simulink library "commblkcod2"  (Simulink 6.0)
settings: Solver=ode45  SolverMode=SingleTasking  StartTime=0.0  StopTime=10.0  RelTol=1e-3
undefined symbols (not defined in the file or in its folder): a, b, G, gfprimfd, k, n, rsgenpoly
libraries: simulink x17, dspsigattribs x17, commblksprivate x6, commutil2 x4, dspmtrx3 x2, commblkcod2 x2
settings Model: RequirementInfo=9  CovMetricSettings=d  Creator=mikem  LastModifiedBy=cvora  ExtModeAutoUpdateStatusClock=off  ProdHWDeviceType=Specified
settings DataIOCC: SignalLoggingName=logsOut
settings OptimizationCC: BooleanDataType=off
settings DebuggingCC: CheckExecutionContextPreStartOutputMsg=on  CheckExecutionContextRuntimeOutputMsg=on  SolverPrmCheckMsg=none
settings HardwareCC: ProdBitPerShort=32  ProdBitPerInt=16  ProdHWDeviceType=Specified  TargetUnknown=on
settings SFSimCC: SFSimApplyToAllLibs=on  SFSimBuildMode=Incremental

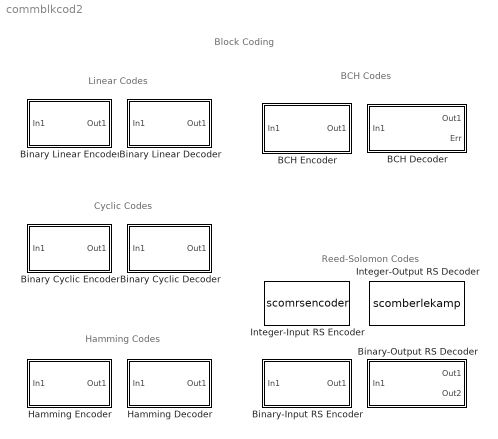
== system commblkcod2 ==
  note: Cyclic Codes
  note: Hamming Codes
  note: BCH Codes
  note: Reed-Solomon Codes
  note: Linear Codes
  note: Block Coding
  BCH Decoder : Subsystem  PropExecContextAcrossSSBoundary=on  mask(BCH Decoder){n=15, k=5, showNumErr=on}
      mask prompts: showNumErr "Output number of corrected errors"
      mask help:
      | Decode a BCH codeword with message length K and codeword length N. N must have the form 2^M-1, where 3 <= M <= 9 .  The values of N and K must produce a valid narrow-sense BCH codeword.
      |
      | The input must contain exactly N elements. The input must be a frame-based column vector.
      mask init:
      | params = commblksbchdec(n,k, showNumErr);
      mask Help: helpview(commbhelp)
      mask Display:
      | plot(0,0,100,100,[5 15 15 5 15 15 5 5 15 15 20 15 75 75 85 75 75 15 75 75 85 85 95 95 85 85 95],[75 75 85 85 85 65 65 95 95 83 80 77 77 73 80 87 83 83 83 87 80 90 90 70 70 80 80]);disp('BCH de');
      | port_label('output',params.portnum, params.portlabel);
  BCH Encoder : Subsystem  PropExecContextAcrossSSBoundary=on  mask(BCH Encoder){n=15, k=5}
      mask help:
      | Create a BCH code with message length K and codeword length N. N must have the form 2^M-1, where 3 <= M <= 9.  The values of N and K must produce a valid narrow-sense BCH codeword.
      |
      | The input must contain exactly K elements. The input must be a frame-based column vector.
      mask init:
      | genpoly = bchgenpoly(n,k);
      | [h, gen] = cyclgen(n,double(genpoly.x));
      | gen1 =[ gen(:,n-k+1:end) gen(:,1:n-k) ];
      mask Help: helpview(commbhelp)
      mask Display: plot(0,0,100,100,[05 15 15 05 05 15 15 15  15 20 15 75 75 85 75 75 15 75 75  85 85 95 95 85 85 95 85 85 95],[80 80 90 90 70 70 90 80  83 80 77 77 73 80 87 83 83 83 87  80 95 95 65 65 85 85 85 75 75]);disp('BCH en')
  Binary Cyclic Decoder : Subsystem  PropExecContextAcrossSSBoundary=on  mask(Binary Cyclic Decoder){n=7, p=4}
      mask prompts: n "Codeword length N:"; p "Message length K, or generator polynomial:"
      mask help:
      | Recover a message vector from a codeword vector of a binary systematic cyclic code.  The message is of length K and the codeword is of length N, where N has the form 2^M-1, for some integer M greater than or equal to 3.
      |
      | The input must contain exactly N elements.  If it is frame-based, then it must be a column vector.
      mask init:
      | m=log2(n+1); if ~isequal(floor(m),m) | n<3,error('N must have the form 2^M-1 for some integer M greater than 2.');end;
      | evalc('if isequal(length(p),1),p=cyclpoly(n,p,''min'');if isempty(p), error(''No cyclic code exists for specified values of N and K.''); end; end;[H,G]=cyclgen(n,p);trt=syndtable(H);');[k,n]=size(G);
      mask Help: helpview(commbhelp)
      mask Display:
      | plot(0,0,100,100,[5 15 15 5 15 15 5 5 15 15 20 15 75 75 85 75 75 15 75 75 85 85 95 95 85 85 95],[75 75 85 85 85 65 65 95 95 83 80 77 77 73 80 87 83 83 83 87 80 90 90 70 70 80 80]);
      | disp('Cyclic de')
  Binary Cyclic Encoder : Subsystem  PropExecContextAcrossSSBoundary=on  mask(Binary Cyclic Encoder){n=7, p=4}
      mask prompts: n "Codeword length N:"; p "Message length K, or generator polynomial:"
      mask help:
      | Create a systematic cyclic code with message length K and codeword length N.  The number N must have the form 2^M-1, where M is an integer greater than or equal to 3.
      |
      | The input must contain exactly K elements.  If it is frame-based, then it must be a column vector.
      mask init:
      | m=log2(n+1); if ~isequal(floor(m),m) | n<3,error('N must have the form 2^M-1 for some integer M >= 3.');end;evalc('if length(p)==1,p=cyclpoly(n,p,''min''); if isempty(p),error(''No cyclic code exists for specified values of N and K.'');end;end;  k=n-length(p)+1; [h,G]=cyclgen(n, p);');
      mask Help: helpview(commbhelp)
      mask Display:
      | plot(0,0,100,100,[05 15 15 05 05 15 15 15  15 20 15 75 75 85 75 75 15 75 75  85 85 95 95 85 85 95 85 85 95],[80 80 90 90 70 70 90 80  83 80 77 77 73 80 87 83 83 83 87  80 95 95 65 65 85 85 85 75 75]);
      | disp('Cyclic en')
  Binary Linear Decoder : Subsystem  PropExecContextAcrossSSBoundary=on  mask(Binary Linear Decoder){G=[[1 1 0; 0 1 1; 1 1 1;1 0 1] eye(4)], trt=0}
      mask prompts: G "Generator matrix (binary K-by-N matrix):"; trt "Decoding table (0 for table corresponding to Generator matrix):"
      mask help:
      | Recover a binary message vector from a binary codeword vector of a linear block code.  The message is of length K and the codeword is of length N, where K and N are the number of rows and columns of the generator matrix respectively.  The number N must have the form 2^M-1, for some integer M greater than or equal to 3.
      |
      | The decoder assumes that the encoder's generator matrix has the standard systematic form [P I].  In other words, the input codewords must contain parity-check bits followed by message bits.
      |
      | The input must contain exactly N elements.  If it is frame-based, then it must be a column vector.
      mask init:
      | [k,n]=size(G);  if k>=n | ~isequal(G(:,n-k+1:n),eye(k)), error('The generator matrix must have the standard systematic form [P I].'); end;
      | H=gen2par(G);if trt==0,evalc('trt=syndtable(H);');end;
      mask Help: helpview(commbhelp)
      mask Display:
      | plot(0,0,100,100,[5 15 15 5 15 15 5 5 15 15 20 15 75 75 85 75 75 15 75 75 85 85 95 95 85 85 95],[75 75 85 85 85 65 65 95 95 83 80 77 77 73 80 87 83 83 83 87 80 90 90 70 70 80 80]);
      | disp('Linear de')
  Binary Linear Encoder : Subsystem  PropExecContextAcrossSSBoundary=on  mask(Binary Linear Encoder){G=[[1 1 0; 0 1 1; 1 1 1; 1 0 1] eye(4)]}
      mask prompts: G "Generator matrix (binary K-by-N matrix):"
      mask help:
      | Create a binary linear block code with message length K and codeword length N, where K and N are the number of rows and columns of the generator matrix respectively.
      |
      | To use the Binary Linear Decoder block at the decoder side, provide a generator matrix in the standard systematic form [P I].
      |
      | The input must contain exactly K elements.  If it is frame-based, then it must be a column vector.
      mask init:
      | [k n]=size(G);
      mask Help: helpview(commbhelp)
      mask Display:
      | plot(0,0,100,100,[05 15 15 05 05 15 15 15  15 20 15 75 75 85 75 75 15 75 75  85 85 95 95 85 85 95 85 85 95],[80 80 90 90 70 70 90 80  83 80 77 77 73 80 87 83 83 83 87  80 95 95 65 65 85 85 85 75 75]);
      | disp('Linear en')
  Binary-Input RS Encoder : Subsystem  PropExecContextAcrossSSBoundary=on  mask(Binary-Input RS Encoder){n=7, k=3, specPrimPoly=off, primPoly=[1 0 1 1], specGenPoly=off, genPoly=rsgenpoly(7,3)}
      mask prompts: n "Codeword length N:"; k "Message length K:"; specPrimPoly "Specify primitive polynomial"; primPoly "Primitive polynomial:"; specGenPoly "Specify generator polynomial"; genPoly "Generator polynomial:"
      mask help:
      | Encode the message in the input vector using an (N,K) Reed-Solomon encoder with the narrow-sense generator polynomial.  The input must be a frame-based column vector with an integer multiple of K*ceil(log2(N+1)) bits.  Each group of K*ceil(log2(N+1)) input bits represents one message word to be encoded.
      |
      | The optional 'Primitive polynomial' parameter is a row vector that represents the binary coefficients of the primitive polynomial in order of descending powers.  When such a user-defined Primitive polynomial is provided, the number of input bits must be an integer multiple of K times the order of the Primitive polynomial instead.
      |
      | The optional 'Generator polynomial' parameter is a row vector that represents the coefficients of the generator polynomial in order of descending powers.  Each coefficient is an element of the Galois field defined by the primitive polynomial.
      mask init:
      | [eStr,params]=commblkrsencbin(gcb, 'init');
      | if(eStr.ecode==1)
      |     error(eStr.emsg);
      | elseif(eStr.ecode==2)
      |     warning(eStr.emsg);
      | end;
      mask Help: helpview(commbhelp)
      mask CallbackString: ||commblkrsencbin(gcb,'cbSpecPrimPoly');||commblkrsencbin(gcb,'cbSpecGenPoly');|
      mask Display:
      | plot(0,0,100,100,[05 15 15 05 05 15 15 15  15 20 15 75 75 85 75 75 15 75 75  85 85 95 95 85 85 95 85 85 95],[80 80 90 90 70 70 90 80  83 80 77 77 73 80 87 83 83 83 87  80 95 95 65 65 85 85 85 75 75]);
      | disp('\nBinary Input\nRS Encoder')
  Binary-Output RS Decoder : Subsystem  PropExecContextAcrossSSBoundary=on  mask(Binary-Output RS Decoder){n=7, k=3, specPrimPoly=off, primPoly=[1 0 1 1], specGenPoly=off, genPoly=rsgenpoly(7,3), showNumErr=on}
      mask prompts: n "Codeword length N:"; k "Message length K:"; specPrimPoly "Specify primitive polynomial"; primPoly "Primitive polynomial:"; specGenPoly "Specify generator polynomial"; genPoly "Generator polynomial:"; showNumErr "Output number of corrected errors"
      mask help:
      | Attempt to decode the input received signal using an (N,K) Reed-Solomon decoder with the narrow-sense generator polynomial.  The input must be a frame-based column vector with an integer multiple of N*ceil(log2(N+1)) bits.  Each group of N*ceil(log2(N+1)) input bits represents one received word to be decoded.
      |
      | The optional 'Primitive polynomial' parameter is a row vector that represents the binary coefficients of the primitive polynomial in order of descending powers.  When such a user-defined Primitive polynomial is provided, the number of input bits must be an integer multiple of N times the order of the Primitive polynomial instead.
      |
      | The optional 'Generator polynomial' parameter is a row vector that represents the coefficients of the generator polynomial in order of descending powers.  Each coefficient is an element of the Galois field defined by the primitive polynomial.
      |
      | The number of corrected errors can be sent to a second output port by checking the 'Output number of corrected errors' check box.  A decoding failure occurs when a certain received word in the input contains more than (N-K)/2 symbol errors.  This is indicated by a value of -1 in the corresponding position in the second output vector.
      mask init:
      | [eStr,params]=commblkrsdecbin(gcb, 'init');
      | if(eStr.ecode==1)
      |     error(eStr.emsg);
      | elseif(eStr.ecode==2)
      |     warning(eStr.emsg);
      | end;
      mask Help: helpview(commbhelp)
      mask CallbackString: ||commblkrsdecbin(gcb,'cbSpecPrimPoly');||commblkrsdecbin(gcb,'cbSpecGenPoly');||commblkrsdecbin(gcb,'cbShowNumErr');
      mask Display:
      | plot(0,0,100,100,[5 15 15 5 15 15 5 5 15 15 20 15 75 75 85 75 75 15 75 75 85 85 95 95 85 85 95],[75 75 85 85 85 65 65 95 95 83 80 77 77 73 80 87 83 83 83 87 80 90 90 70 70 80 80]);
      | disp('\nBinary Output\nRS Decoder')
      | text(params.x,params.y,params.portlabel)
  Hamming Decoder : Subsystem  PropExecContextAcrossSSBoundary=on  mask(Hamming Decoder){n=7, k=gfprimfd(3,'min')}
      mask prompts: n "Codeword length N:"; k "Message length K, or M-degree primitive polynomial:"
      mask help:
      | Recover a binary message vector from a binary Hamming codeword vector.  The message is of length K and the codeword is of length N, where N has the form 2^M-1, for some integer M greater than or equal to 3.  K must equal N-M.
      |
      | The input must contain exactly N elements.  If it is frame-based, then it must be a column vector.
      mask init:
      | if length(k)>1,p=k;k=n-length(p)+1;
      | else,evalc('p=gfprimdf(n-k);');end;
      | m=log2(n+1);if ~isequal(floor(m),m) | ~isequal(n-k,m), error('N must have the form 2^M-1 where M is an integer >=3.  K must equal N-M.');end;
      | evalc('[H,G]=hammgen(n-k,p);trt=syndtable(H);');[a,b]=size(G);
      mask Help: helpview(commbhelp)
      mask Display: plot(0,0,100,100,[1 3 3 1 3 3 1 1 3 3 4 3 15 15 17 15 15 3 15 15 17 17 19 19 17 17 19]*5,[-5 -5 5 5 5 -15 -15 15 15 3 0 -3 -3 -7 0 7 3 3 3 7 0 10 10 -10 -10 0 0]+80);disp('Hamming de')
  Hamming Encoder : Subsystem  PropExecContextAcrossSSBoundary=on  mask(Hamming Encoder){n=7, k=gfprimfd(3,'min')}
      mask prompts: n "Codeword length N:"; k "Message length K, or M-degree primitive polynomial:"
      mask help:
      | Create a Hamming code with message length K and codeword length N.  The number N must have the form 2^M-1, where M is an integer greater than or equal to 3.  K must equal N-M.
      |
      | The input must contain exactly K elements.  If it is frame-based, then it must be a column vector.
      mask init:
      | if length(k)>1, p=k; k=n-length(k)+1;
      | else, evalc('p=gfprimdf(n-k);'); end;
      | m=log2(n+1);if ~isequal(floor(m),m) | ~isequal(n-k,m), error('N must have the form 2^M-1 where M is an integer >=3.  K must equal N-M.');end;
      | evalc('[h,G]=hammgen(n-k,p);');
      mask Help: helpview(commbhelp)
      mask Display: plot(0,0,100,100,[1 3 3 1 1 3 3 3 3 4 3 15 15 17 15 15 3 15 15 17 17 19 19 17 17 19 17 17 19]*5,[0 0 10 10 -10 -10 10 0 3 0 -3 -3 -7 0 7 3 3 3 7 0 15 15 -15 -15 5 5 5 -5 -5]+80);disp('Hamming en')
  Integer-Input RS Encoder : S-Function  FunctionName=scomrsencoder  Parameters=n, k, params.m, params.primPoly, params.genPoly, params.shortened  mask(Integer-Input RS Encoder){n=7, k=3, specPrimPoly=off, primPoly=[1 0 1 1], specGenPoly=off, genPoly=rsgenpoly(7,3)}
      mask prompts: n "Codeword length N:"; k "Message length K:"; specPrimPoly "Specify primitive polynomial"; primPoly "Primitive polynomial:"; specGenPoly "Specify generator polynomial"; genPoly "Generator polynomial:"
      mask help:
      | Encode the message in the input vector using an (N,K) Reed-Solomon encoder with the narrow-sense generator polynomial.  The input must be a frame-based column vector with an integer multiple of K elements.  Each group of K input elements represents one message word to be encoded.  Each symbol must have ceil(log2(N+1)) bits.
      |
      | The optional 'Primitive polynomial' parameter is a row vector that represents the binary coefficients of the primitive polynomial in order of descending powers.  When such a user-defined Primitive polynomial is provided, the number of bits in each input symbol must equal the order of the Primitive polynomial instead.
      |
      | The optional 'Generator polynomial' parameter is a row vector that represents the coefficients of the generator polynomial in order of descending powers.  Each coefficient is an element of the Galois field defined by the primtive polynomial.
      mask init:
      | [eStr,params]=commblkrsencoder(gcb, 'init');
      | if(eStr.ecode==1)
      |     error(eStr.emsg);
      | elseif(eStr.ecode==2)
      |     warning(eStr.emsg);
      | end;
      mask Help: helpview(commbhelp)
      mask CallbackString: ||commblkrsencoder(gcb,'cbSpecPrimPoly');||commblkrsencoder(gcb,'cbSpecGenPoly');|
      mask Display:
      | plot(0,0,100,100,[05 15 15 05 05 15 15 15  15 20 15 75 75 85 75 75 15 75 75  85 85 95 95 85 85 95 85 85 95],[80 80 90 90 70 70 90 80  83 80 77 77 73 80 87 83 83 83 87  80 95 95 65 65 85 85 85 75 75]);
      | disp('\nRS Encoder')
  Integer-Output RS Decoder : S-Function  FunctionName=scomberlekamp  Parameters=n, k, params.m, params.t, params.primPoly, params.b, params.shortened, showNumErr  mask(Integer-Output RS Decoder){n=7, k=3, specPrimPoly=off, primPoly=[1 0 1 1], specGenPoly=off, genPoly=rsgenpoly(7,3), showNumErr=on}
      mask prompts: n "Codeword length N:"; k "Message length K:"; specPrimPoly "Specify primitive polynomial"; primPoly "Primitive polynomial:"; specGenPoly "Specify generator polynomial"; genPoly "Generator polynomial:"; showNumErr "Output number of corrected errors"
      mask help:
      | Attempt to decode the input received signal using an (N,K) Reed-Solomon decoder with the narrow-sense generator polynomial.  The input must be a frame-based column vector with an integer multiple of N elements.  Each group of N input elements represents one received word to be decoded.  Each symbol must have ceil(log2(N+1)) bits.
      |
      | The optional 'Primitive polynomial' parameter is a row vector that represents the binary coefficients of the primitive polynomial in order of descending powers.  When such a user-defined Primitive polynomial is provided, the number of bits in each input symbol must equal the order of the Primitive polynomial instead.
      |
      | The optional 'Generator polynomial' parameter is a row vector that represents the coefficients of the generator polynomial in order of descending powers.  Each coefficient is an element of the Galois field defined by the primitive polynomial.
      |
      | The number of corrected errors can be sent to a second output port by checking the 'Output number of corrected errors' check box.  A decoding failure occurs when a certain word in the input contains more than (N-K)/2 errors.  This is indicated by a value of -1 in the corresponding position in the second output vector.
      mask init:
      | [eStr,params]=commblkrsdecoder(gcb, 'init');
      | if(eStr.ecode==1)
      |     error(eStr.emsg);
      | elseif(eStr.ecode==2)
      |     warning(eStr.emsg);
      | end;
      mask Help: helpview(commbhelp)
      mask CallbackString: ||commblkrsdecoder(gcb,'cbSpecPrimPoly');||commblkrsdecoder(gcb,'cbSpecGenPoly');||
      mask Display:
      | plot(0,0,100,100,[5 15 15 5 15 15 5 5 15 15 20 15 75 75 85 75 75 15 75 75 85 85 95 95 85 85 95],[75 75 85 85 85 65 65 95 95 83 80 77 77 73 80 87 83 83 83 87 80 90 90 70 70 80 80]);
      | disp('\nRS Decoder')
      | port_label('output',params.portnum,params.portlabel);

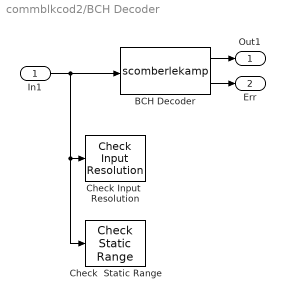
== system commblkcod2/BCH Decoder ==
  In1 : Inport  LatchInput=off
  BCH Decoder : S-Function  FunctionName=scomberlekamp  Parameters=n,k,params.m, params.t,params.poly,1,0,1
  Check  Static Range : simulink/Model Verification/Check  Static Range  Description=0 <= u <= 1  max=1  max_included=on  min=0  min_included=on  enabled=on  callback=error('Input must be 0 or 1')  stopWhenAssertionFail=on  export=off  icon=graphic
  Check Input  Resolution : simulink/Model Verification/Check Input  Resolution  Description=-Inf < u < +Inf  resolution=1  enabled=on  callback=error('Input must be 0 or 1')  stopWhenAssertionFail=on  export=off
  Out1 : Outport
  Err : Outport  Port=2
  wires:
  BCH Decoder/2 -> Err/1
  BCH Decoder/1 -> Out1/1
  In1/1 -> BCH Decoder/1, Check Input  Resolution/1, Check  Static Range/1

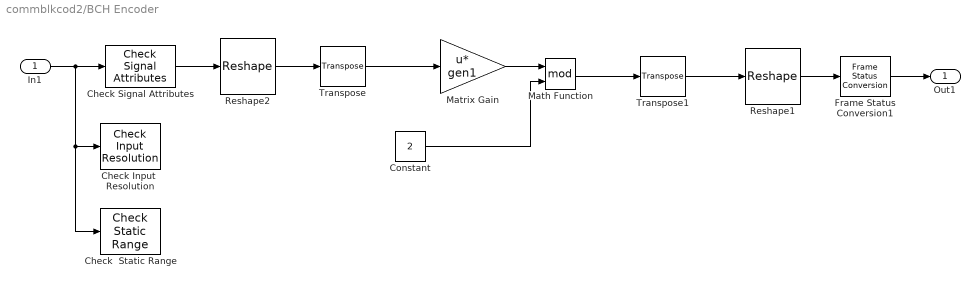
== system commblkcod2/BCH Encoder ==
  In1 : Inport  LatchInput=off
  Check  Static Range : simulink/Model Verification/Check  Static Range  Description=0 <= u <= 1  max=1  max_included=on  min=0  min_included=on  enabled=on  callback=error('Input must be 0 or 1')  stopWhenAssertionFail=on  export=off  icon=graphic
  Check Input  Resolution : simulink/Model Verification/Check Input  Resolution  Description=-Inf < u < +Inf  resolution=1  enabled=on  callback=error('Input must be 0 or 1')  stopWhenAssertionFail=on  export=off
  Check Signal Attributes : dspsigattribs/Check Signal Attributes  SigAttribCheckMethod=Does not match attributes exactly  Complexity=Real  Frame=Frame-based  DimsCheckMethod=Is...  Dimensions=Column vector (2-D)  DatatypeCheckMethod=Ignore  DatatypeGeneral=Boolean  DtypeFloatSpecific=Any floating-point  DtypeFixedSpecific=Any fixed-point  DtypeIntSpecific=Any integer  SampleMode=Ignore
      settings: AttributesFormatString=\n
  Constant : Constant  Value=2
  Frame Status Conversion1 : dspsigattribs/Frame Status Conversion  growRefPort=off  outframe=Frame-based
      settings: AttributesFormatString=\n
  Math Function : Math  Operator=mod  SaturateOnIntegerOverflow=on
  Matrix Gain : Gain  Gain=gen1  Multiplication=Matrix(u*K)  SaturateOnIntegerOverflow=on
  Reshape1 : simulink/Math Operations/Reshape  OutputDimensionality=Customize  OutputDimensions=[n,1]
  Reshape2 : simulink/Math Operations/Reshape  OutputDimensionality=Customize  OutputDimensions=[k, 1 ]
  Transpose : dspmtrx3/Transpose  Hermitian=off
      settings: AttributesFormatString=\n
  Transpose1 : dspmtrx3/Transpose  Hermitian=off
      settings: AttributesFormatString=\n
  Out1 : Outport
  wires:
  Check Signal Attributes/1 -> Reshape2/1
  Frame Status Conversion1/1 -> Out1/1
  Reshape1/1 -> Frame Status Conversion1/1
  Transpose1/1 -> Reshape1/1
  Transpose/1 -> Matrix Gain/1
  In1/1 -> Check Signal Attributes/1, Check Input  Resolution/1, Check  Static Range/1
  Math Function/1 -> Transpose1/1
  Reshape2/1 -> Transpose/1
  Constant/1 -> Math Function/2
  Matrix Gain/1 -> Math Function/1

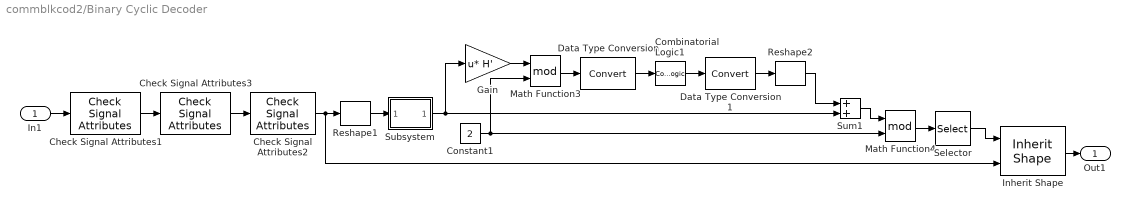
== system commblkcod2/Binary Cyclic Decoder ==
  In1 : Inport  LatchInput=off
  Check Signal Attributes1 : dspsigattribs/Check Signal Attributes  SigAttribCheckMethod=Matches attributes exactly  Complexity=Ignore  Frame=Frame-based  DimsCheckMethod=Is...  Dimensions=Row vector (2-D)  DatatypeCheckMethod=Ignore  DatatypeGeneral=Boolean  DtypeFloatSpecific=Any floating-point  DtypeFixedSpecific=Any fixed-point  DtypeIntSpecific=Any integer  SampleMode=Ignore
  Check Signal Attributes2 : dspsigattribs/Check Signal Attributes  SigAttribCheckMethod=Matches attributes exactly  Complexity=Ignore  Frame=Ignore  DimsCheckMethod=Is...  Dimensions=Full matrix (2-D)  DatatypeCheckMethod=Ignore  DatatypeGeneral=Boolean  DtypeFloatSpecific=Any floating-point  DtypeFixedSpecific=Any fixed-point  DtypeIntSpecific=Any integer  SampleMode=Ignore
  Check Signal Attributes3 : dspsigattribs/Check Signal Attributes  SigAttribCheckMethod=Matches attributes exactly  Complexity=Ignore  Frame=Ignore  DimsCheckMethod=Is...  Dimensions=Scalar (1-D or 2-D)  DatatypeCheckMethod=Ignore  DatatypeGeneral=Boolean  DtypeFloatSpecific=Any floating-point  DtypeFixedSpecific=Any fixed-point  DtypeIntSpecific=Any integer  SampleMode=Ignore
  Combinatorial Logic1 : CombinatorialLogic  TruthTable=trt
  Constant1 : Constant  Value=2
  Data Type Conversion : DataTypeConversion  OutDataTypeMode=boolean  SaturateOnIntegerOverflow=on  RndMeth=Zero
  Data Type Conversion1 : DataTypeConversion  OutDataTypeMode=double  SaturateOnIntegerOverflow=on  RndMeth=Zero
  Gain : Gain  Gain=H'  Multiplication=Matrix(u*K)  SaturateOnIntegerOverflow=on
  Inherit Shape : commblksprivate/Inherit Shape
  Math Function3 : Math  Operator=mod  SaturateOnIntegerOverflow=on
  Math Function4 : Math  Operator=mod  SaturateOnIntegerOverflow=on
  Reshape1 : simulink/Math Operations/Reshape  OutputDimensionality=Row vector  OutputDimensions=[1,1]
  Reshape2 : simulink/Math Operations/Reshape  OutputDimensionality=Row vector  OutputDimensions=[1,1]
  Selector : Selector  Elements=[n-k+1:n]  InputPortWidth=n
  Subsystem : Subsystem  AncestorBlock=commblkcod2/Binary Linear Decoder/Subsystem  PropExecContextAcrossSSBoundary=on
  Sum1 : Sum  SaturateOnIntegerOverflow=on  InputSameDT=on
  Out1 : Outport
  wires:
  Check Signal Attributes1/1 -> Check Signal Attributes3/1
  Check Signal Attributes2/1 -> Reshape1/1, Inherit Shape/2
  Inherit Shape/1 -> Out1/1
  In1/1 -> Check Signal Attributes1/1
  Gain/1 -> Math Function3/1
  Combinatorial Logic1/1 -> Data Type Conversion1/1
  Sum1/1 -> Math Function4/1
  Math Function4/1 -> Selector/1
  Math Function3/1 -> Data Type Conversion/1
  Constant1/1 -> Math Function3/2, Math Function4/2
  Selector/1 -> Inherit Shape/1
  Reshape1/1 -> Subsystem/1(In1)
  Subsystem/1(Out1) -> Gain/1, Sum1/2
  Check Signal Attributes3/1 -> Check Signal Attributes2/1
  Reshape2/1 -> Sum1/1
  Data Type Conversion1/1 -> Reshape2/1
  Data Type Conversion/1 -> Combinatorial Logic1/1

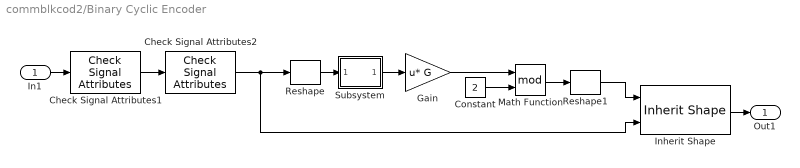
== system commblkcod2/Binary Cyclic Encoder ==
  In1 : Inport  LatchInput=off
  Check Signal Attributes1 : dspsigattribs/Check Signal Attributes  SigAttribCheckMethod=Matches attributes exactly  Complexity=Ignore  Frame=Frame-based  DimsCheckMethod=Is...  Dimensions=Row vector (2-D)  DatatypeCheckMethod=Ignore  DatatypeGeneral=Boolean  DtypeFloatSpecific=Any floating-point  DtypeFixedSpecific=Any fixed-point  DtypeIntSpecific=Any integer  SampleMode=Ignore
  Check Signal Attributes2 : dspsigattribs/Check Signal Attributes  SigAttribCheckMethod=Matches attributes exactly  Complexity=Ignore  Frame=Ignore  DimsCheckMethod=Is...  Dimensions=Full matrix (2-D)  DatatypeCheckMethod=Ignore  DatatypeGeneral=Boolean  DtypeFloatSpecific=Any floating-point  DtypeFixedSpecific=Any fixed-point  DtypeIntSpecific=Any integer  SampleMode=Ignore
  Constant : Constant  Value=2
  Gain : Gain  Gain=G  Multiplication=Matrix(u*K)  SaturateOnIntegerOverflow=on
  Inherit Shape : commblksprivate/Inherit Shape
  Math Function : Math  Operator=mod  SaturateOnIntegerOverflow=on
  Reshape : simulink/Math Operations/Reshape  OutputDimensionality=Row vector  OutputDimensions=[1,1]
  Reshape1 : simulink/Math Operations/Reshape  OutputDimensionality=Column vector  OutputDimensions=[1,1]
  Subsystem : Subsystem  AncestorBlock=commblkcod2/Binary Linear Decoder/Subsystem  PropExecContextAcrossSSBoundary=on
  Out1 : Outport
  wires:
  Constant/1 -> Math Function/2
  Gain/1 -> Math Function/1
  Check Signal Attributes1/1 -> Check Signal Attributes2/1
  Check Signal Attributes2/1 -> Reshape/1, Inherit Shape/2
  Math Function/1 -> Reshape1/1
  Reshape/1 -> Subsystem/1(In1)
  In1/1 -> Check Signal Attributes1/1
  Inherit Shape/1 -> Out1/1
  Subsystem/1(Out1) -> Gain/1
  Reshape1/1 -> Inherit Shape/1

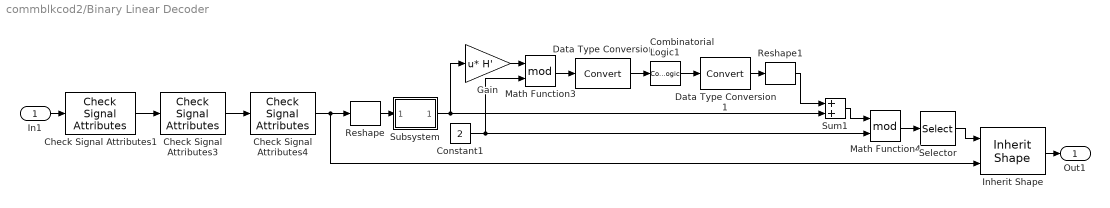
== system commblkcod2/Binary Linear Decoder ==
  In1 : Inport  LatchInput=off
  Check Signal Attributes1 : dspsigattribs/Check Signal Attributes  SigAttribCheckMethod=Matches attributes exactly  Complexity=Ignore  Frame=Frame-based  DimsCheckMethod=Is...  Dimensions=Row vector (2-D)  DatatypeCheckMethod=Ignore  DatatypeGeneral=Boolean  DtypeFloatSpecific=Any floating-point  DtypeFixedSpecific=Any fixed-point  DtypeIntSpecific=Any integer  SampleMode=Ignore
  Check Signal Attributes3 : dspsigattribs/Check Signal Attributes  SigAttribCheckMethod=Matches attributes exactly  Complexity=Ignore  Frame=Ignore  DimsCheckMethod=Is...  Dimensions=Scalar (1-D or 2-D)  DatatypeCheckMethod=Ignore  DatatypeGeneral=Boolean  DtypeFloatSpecific=Any floating-point  DtypeFixedSpecific=Any fixed-point  DtypeIntSpecific=Any integer  SampleMode=Ignore
  Check Signal Attributes4 : dspsigattribs/Check Signal Attributes  SigAttribCheckMethod=Matches attributes exactly  Complexity=Ignore  Frame=Ignore  DimsCheckMethod=Is...  Dimensions=Full matrix (2-D)  DatatypeCheckMethod=Ignore  DatatypeGeneral=Boolean  DtypeFloatSpecific=Any floating-point  DtypeFixedSpecific=Any fixed-point  DtypeIntSpecific=Any integer  SampleMode=Ignore
  Combinatorial Logic1 : CombinatorialLogic  TruthTable=trt
  Constant1 : Constant  Value=2
  Data Type Conversion : DataTypeConversion  OutDataTypeMode=boolean  SaturateOnIntegerOverflow=on  RndMeth=Zero
  Data Type Conversion1 : DataTypeConversion  OutDataTypeMode=double  SaturateOnIntegerOverflow=on  RndMeth=Zero
  Gain : Gain  Gain=H'  Multiplication=Matrix(u*K)  SaturateOnIntegerOverflow=on
  Inherit Shape : commblksprivate/Inherit Shape
  Math Function3 : Math  Operator=mod  SaturateOnIntegerOverflow=on
  Math Function4 : Math  Operator=mod  SaturateOnIntegerOverflow=on
  Reshape : simulink/Math Operations/Reshape  OutputDimensionality=Row vector  OutputDimensions=[1,1]
  Reshape1 : simulink/Math Operations/Reshape  OutputDimensionality=Row vector  OutputDimensions=[1,1]
  Selector : Selector  Elements=[n-k+1:n]  InputPortWidth=n
  Subsystem : Subsystem  AncestorBlock=commblkcod2/Binary Linear Encoder/Subsystem  PropExecContextAcrossSSBoundary=on
  Sum1 : Sum  SaturateOnIntegerOverflow=on  InputSameDT=on
  Out1 : Outport
  wires:
  Gain/1 -> Math Function3/1
  Combinatorial Logic1/1 -> Data Type Conversion1/1
  Sum1/1 -> Math Function4/1
  Math Function4/1 -> Selector/1
  Math Function3/1 -> Data Type Conversion/1
  Constant1/1 -> Math Function4/2, Math Function3/2
  In1/1 -> Check Signal Attributes1/1
  Check Signal Attributes1/1 -> Check Signal Attributes3/1
  Selector/1 -> Inherit Shape/1
  Reshape/1 -> Subsystem/1(In1)
  Subsystem/1(Out1) -> Sum1/2, Gain/1
  Inherit Shape/1 -> Out1/1
  Check Signal Attributes3/1 -> Check Signal Attributes4/1
  Check Signal Attributes4/1 -> Reshape/1, Inherit Shape/2
  Reshape1/1 -> Sum1/1
  Data Type Conversion/1 -> Combinatorial Logic1/1
  Data Type Conversion1/1 -> Reshape1/1

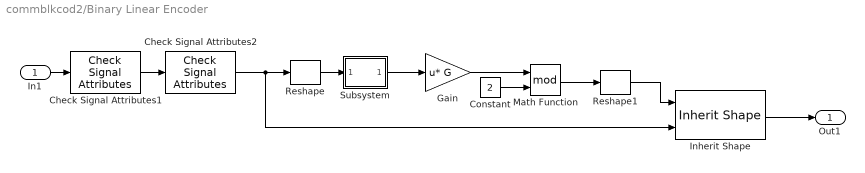
== system commblkcod2/Binary Linear Encoder ==
  In1 : Inport  LatchInput=off
  Check Signal Attributes1 : dspsigattribs/Check Signal Attributes  SigAttribCheckMethod=Matches attributes exactly  Complexity=Ignore  Frame=Frame-based  DimsCheckMethod=Is...  Dimensions=Row vector (2-D)  DatatypeCheckMethod=Ignore  DatatypeGeneral=Boolean  DtypeFloatSpecific=Any floating-point  DtypeFixedSpecific=Any fixed-point  DtypeIntSpecific=Any integer  SampleMode=Ignore
  Check Signal Attributes2 : dspsigattribs/Check Signal Attributes  SigAttribCheckMethod=Matches attributes exactly  Complexity=Ignore  Frame=Ignore  DimsCheckMethod=Is...  Dimensions=Full matrix (2-D)  DatatypeCheckMethod=Ignore  DatatypeGeneral=Boolean  DtypeFloatSpecific=Any floating-point  DtypeFixedSpecific=Any fixed-point  DtypeIntSpecific=Any integer  SampleMode=Ignore
  Constant : Constant  Value=2
  Gain : Gain  Gain=G  Multiplication=Matrix(u*K)  SaturateOnIntegerOverflow=on
  Inherit Shape : commblksprivate/Inherit Shape
  Math Function : Math  Operator=mod  SaturateOnIntegerOverflow=on
  Reshape : simulink/Math Operations/Reshape  OutputDimensionality=Row vector  OutputDimensions=[1,1]
  Reshape1 : simulink/Math Operations/Reshape  OutputDimensionality=Column vector  OutputDimensions=[1,1]
  Subsystem : Subsystem  AncestorBlock=commblkcod2/Binary Linear Decoder/Subsystem  PropExecContextAcrossSSBoundary=on
  Out1 : Outport
  wires:
  Constant/1 -> Math Function/2
  In1/1 -> Check Signal Attributes1/1
  Check Signal Attributes1/1 -> Check Signal Attributes2/1
  Check Signal Attributes2/1 -> Inherit Shape/2, Reshape/1
  Math Function/1 -> Reshape1/1
  Inherit Shape/1 -> Out1/1
  Reshape/1 -> Subsystem/1(In1)
  Gain/1 -> Math Function/1
  Subsystem/1(Out1) -> Gain/1
  Reshape1/1 -> Inherit Shape/1

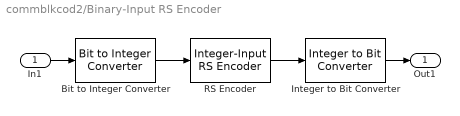
== system commblkcod2/Binary-Input RS Encoder ==
  In1 : Inport  LatchInput=off
  Bit to Integer Converter : commutil2/Bit to Integer Converter  nbits=params.m
  Integer to Bit Converter : commutil2/Integer to Bit Converter  nbits=params.m
  RS Encoder : commblkcod2/Integer-Input RS Encoder  n=n  k=k  specPrimPoly=off  primPoly=primPoly  specGenPoly=off  genPoly=genPoly
  Out1 : Outport
  wires:
  Bit to Integer Converter/1 -> RS Encoder/1
  RS Encoder/1 -> Integer to Bit Converter/1
  Integer to Bit Converter/1 -> Out1/1
  In1/1 -> Bit to Integer Converter/1

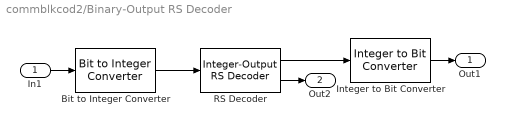
== system commblkcod2/Binary-Output RS Decoder ==
  In1 : Inport  LatchInput=off
  Bit to Integer Converter : commutil2/Bit to Integer Converter  nbits=params.m
  Integer to Bit Converter : commutil2/Integer to Bit Converter  nbits=params.m
  RS Decoder : commblkcod2/Integer-Output RS Decoder  n=n  k=k  specPrimPoly=off  primPoly=primPoly  specGenPoly=off  genPoly=genPoly  showNumErr=on
  Out1 : Outport
  Out2 : Outport  Port=2
  wires:
  In1/1 -> Bit to Integer Converter/1
  Integer to Bit Converter/1 -> Out1/1
  Bit to Integer Converter/1 -> RS Decoder/1
  RS Decoder/1 -> Integer to Bit Converter/1
  RS Decoder/2 -> Out2/1

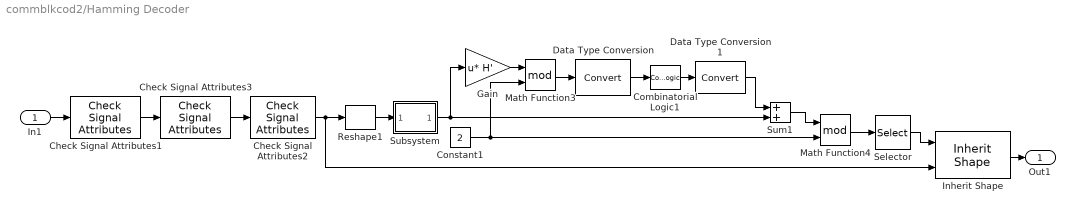
== system commblkcod2/Hamming Decoder ==
  In1 : Inport  LatchInput=off
  Check Signal Attributes1 : dspsigattribs/Check Signal Attributes  SigAttribCheckMethod=Matches attributes exactly  Complexity=Ignore  Frame=Frame-based  DimsCheckMethod=Is...  Dimensions=Row vector (2-D)  DatatypeCheckMethod=Ignore  DatatypeGeneral=Boolean  DtypeFloatSpecific=Any floating-point  DtypeFixedSpecific=Any fixed-point  DtypeIntSpecific=Any integer  SampleMode=Ignore
  Check Signal Attributes2 : dspsigattribs/Check Signal Attributes  SigAttribCheckMethod=Matches attributes exactly  Complexity=Ignore  Frame=Ignore  DimsCheckMethod=Is...  Dimensions=Full matrix (2-D)  DatatypeCheckMethod=Ignore  DatatypeGeneral=Boolean  DtypeFloatSpecific=Any floating-point  DtypeFixedSpecific=Any fixed-point  DtypeIntSpecific=Any integer  SampleMode=Ignore
  Check Signal Attributes3 : dspsigattribs/Check Signal Attributes  SigAttribCheckMethod=Matches attributes exactly  Complexity=Ignore  Frame=Ignore  DimsCheckMethod=Is...  Dimensions=Scalar (1-D or 2-D)  DatatypeCheckMethod=Ignore  DatatypeGeneral=Boolean  DtypeFloatSpecific=Any floating-point  DtypeFixedSpecific=Any fixed-point  DtypeIntSpecific=Any integer  SampleMode=Ignore
  Combinatorial Logic1 : CombinatorialLogic  TruthTable=trt
  Constant1 : Constant  Value=2
  Data Type Conversion : DataTypeConversion  OutDataTypeMode=boolean  SaturateOnIntegerOverflow=on  RndMeth=Zero
  Data Type Conversion1 : DataTypeConversion  OutDataTypeMode=double  SaturateOnIntegerOverflow=on  RndMeth=Zero
  Gain : Gain  Gain=H'  Multiplication=Matrix(u*K)  SaturateOnIntegerOverflow=on
  Inherit Shape : commblksprivate/Inherit Shape
  Math Function3 : Math  Operator=mod  SaturateOnIntegerOverflow=on
  Math Function4 : Math  Operator=mod  SaturateOnIntegerOverflow=on
  Reshape1 : simulink/Math Operations/Reshape  OutputDimensionality=Row vector  OutputDimensions=[1,1]
  Selector : Selector  Elements=[b-a+1:b]  InputPortWidth=b
  Subsystem : Subsystem  AncestorBlock=commblkcod2/Binary Linear Decoder/Subsystem  PropExecContextAcrossSSBoundary=on
  Sum1 : Sum  SaturateOnIntegerOverflow=on  InputSameDT=on
  Out1 : Outport
  wires:
  In1/1 -> Check Signal Attributes1/1
  Check Signal Attributes1/1 -> Check Signal Attributes3/1
  Check Signal Attributes2/1 -> Reshape1/1, Inherit Shape/2
  Gain/1 -> Math Function3/1
  Combinatorial Logic1/1 -> Data Type Conversion1/1
  Sum1/1 -> Math Function4/1
  Math Function4/1 -> Selector/1
  Math Function3/1 -> Data Type Conversion/1
  Constant1/1 -> Math Function4/2, Math Function3/2
  Selector/1 -> Inherit Shape/1
  Reshape1/1 -> Subsystem/1(In1)
  Subsystem/1(Out1) -> Sum1/2, Gain/1
  Inherit Shape/1 -> Out1/1
  Check Signal Attributes3/1 -> Check Signal Attributes2/1
  Data Type Conversion/1 -> Combinatorial Logic1/1
  Data Type Conversion1/1 -> Sum1/1

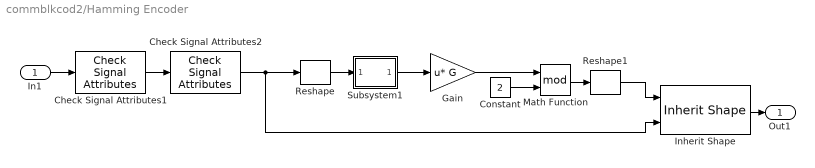
== system commblkcod2/Hamming Encoder ==
  In1 : Inport  LatchInput=off
  Check Signal Attributes1 : dspsigattribs/Check Signal Attributes  SigAttribCheckMethod=Matches attributes exactly  Complexity=Ignore  Frame=Frame-based  DimsCheckMethod=Is...  Dimensions=Row vector (2-D)  DatatypeCheckMethod=Ignore  DatatypeGeneral=Boolean  DtypeFloatSpecific=Any floating-point  DtypeFixedSpecific=Any fixed-point  DtypeIntSpecific=Any integer  SampleMode=Ignore
  Check Signal Attributes2 : dspsigattribs/Check Signal Attributes  SigAttribCheckMethod=Matches attributes exactly  Complexity=Ignore  Frame=Ignore  DimsCheckMethod=Is...  Dimensions=Full matrix (2-D)  DatatypeCheckMethod=Ignore  DatatypeGeneral=Boolean  DtypeFloatSpecific=Any floating-point  DtypeFixedSpecific=Any fixed-point  DtypeIntSpecific=Any integer  SampleMode=Ignore
  Constant : Constant  Value=2
  Gain : Gain  Gain=G  Multiplication=Matrix(u*K)  SaturateOnIntegerOverflow=on
  Inherit Shape : commblksprivate/Inherit Shape
  Math Function : Math  Operator=mod  SaturateOnIntegerOverflow=on
  Reshape : simulink/Math Operations/Reshape  OutputDimensionality=Row vector  OutputDimensions=[1,1]
  Reshape1 : simulink/Math Operations/Reshape  OutputDimensionality=Column vector  OutputDimensions=[1,1]
  Subsystem1 : Subsystem  AncestorBlock=commblkcod2/Binary Linear Decoder/Subsystem  PropExecContextAcrossSSBoundary=on
  Out1 : Outport
  wires:
  Constant/1 -> Math Function/2
  Gain/1 -> Math Function/1
  Check Signal Attributes1/1 -> Check Signal Attributes2/1
  Check Signal Attributes2/1 -> Inherit Shape/2, Reshape/1
  Math Function/1 -> Reshape1/1
  Reshape/1 -> Subsystem1/1(In1)
  In1/1 -> Check Signal Attributes1/1
  Inherit Shape/1 -> Out1/1
  Subsystem1/1(Out1) -> Gain/1
  Reshape1/1 -> Inherit Shape/1

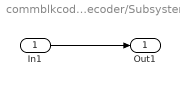
== system commblkcod2/Binary Cyclic Decoder/Subsystem ==
  In1 : Inport  PortDimensions=[1 n]  LatchInput=off
  Out1 : Outport
  wires:
  In1/1 -> Out1/1

== system commblkcod2/Binary Cyclic Encoder/Subsystem ==
  In1 : Inport  PortDimensions=[1 k]  LatchInput=off
  Out1 : Outport
  wires:
  In1/1 -> Out1/1

== system commblkcod2/Binary Linear Decoder/Subsystem ==
  In1 : Inport  PortDimensions=[1 n]  LatchInput=off
  Out1 : Outport
  wires:
  In1/1 -> Out1/1

== system commblkcod2/Binary Linear Encoder/Subsystem ==
  In1 : Inport  PortDimensions=[1 k]  LatchInput=off
  Out1 : Outport
  wires:
  In1/1 -> Out1/1

== system commblkcod2/Hamming Decoder/Subsystem ==
  In1 : Inport  PortDimensions=[1 n]  LatchInput=off
  Out1 : Outport
  wires:
  In1/1 -> Out1/1

== system commblkcod2/Hamming Encoder/Subsystem1 ==
  In1 : Inport  PortDimensions=[1 k]  LatchInput=off
  Out1 : Outport
  wires:
  In1/1 -> Out1/1
